simulink model "interpretar_ensaios"  (R2012b)
settings: Solver=ode3  StartTime=0.0  StopTime=4.9999  FixedStep=1e-4  MaxStep=1e-4  RelTol=1e-3
libraries: simulink x3, Encoder x1
settings Model: Creator=h3now  LastModifiedBy=h3now

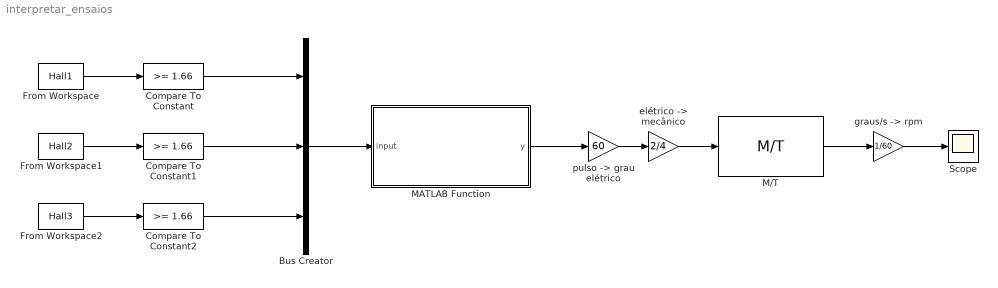
== system interpretar_ensaios ==
  Bus Creator : BusCreator  Inputs=3
  Compare To Constant : simulink/Logic and Bit Operations/Compare To Constant  relop=>=  const=1.66  OutDataTypeStr=uint8
  Compare To Constant1 : simulink/Logic and Bit Operations/Compare To Constant  relop=>=  const=1.66  OutDataTypeStr=uint8
  Compare To Constant2 : simulink/Logic and Bit Operations/Compare To Constant  relop=>=  const=1.66  OutDataTypeStr=uint8
  From Workspace : FromWorkspace  VariableName=Hall1  SampleTime=0  OutputAfterFinalValue=Holding final value
  From Workspace1 : FromWorkspace  VariableName=Hall2  SampleTime=0
  From Workspace2 : FromWorkspace  VariableName=Hall3  SampleTime=0
  M/T : Encoder/M//T  Ts=0.01
  MATLAB Function : MATLAB Function  TreatAsAtomicUnit=on
  Scope : Scope
      settings: SaveName=vel  SampleInput=on
  "elétrico -> mecânico" : Gain  Gain=2/4
  "graus/s -> rpm" : Gain  Gain=1/60
  "pulso -> grau elétrico" : Gain  Gain=60
  wires:
  Bus Creator/1 -> MATLAB Function/1(input)
  From Workspace/1 -> Compare To Constant/1
  From Workspace1/1 -> Compare To Constant1/1
  From Workspace2/1 -> Compare To Constant2/1
  Compare To Constant/1 -> Bus Creator/1
  Compare To Constant1/1 -> Bus Creator/2
  Compare To Constant2/1 -> Bus Creator/3
  MATLAB Function/1(y) -> "pulso -> grau elétrico"/1
  "pulso -> grau elétrico"/1 -> "elétrico -> mecânico"/1
  "elétrico -> mecânico"/1 -> M/T/1
  M/T/1 -> "graus/s -> rpm"/1
  "graus/s -> rpm"/1 -> Scope/1

== matlab function interpretar_ensaios/MATLAB Function ==
  data: y output; input input
function y = state_machine(input)
%#codegen

% Initializing persistent variables.
persistent theta;
persistent state;
if isempty(theta)
    % 'theta' stores the angular position.
    theta = 0; 
    
    % check starting state and store it in 'state'.
    if isequal(input, [0,0,1]')
        state = 0;
    elseif isequal(input, [1,0,1]')
        state = 1;
    elseif isequal(input, [1,0,0]')
        state = 2;
    elseif isequal(input, [1,1,0]')
        state = 3;
    elseif isequal(input, [0,1,0]')
        state = 4;
    elseif isequal(input, [0,1,1]')
        state = 5;
    else
        state = -1;
    end
        
end

% State machine.
switch state
    case 0
        % keep state.
        if isequal(input,[0,0,1]')
        % go to next state.
        elseif isequal(input,[1,0,1]')
            state = 1;
            theta = theta + 1;
        % go to previous state.
        elseif isequal(input,[0,1,1]')
            state = 5;
            theta = theta - 1;
        % go to error state.
        else
            state = -1;
        end
        
    case 1
        % keep state.
        if isequal(input,[1,0,1]')
        % go to next state.
        elseif isequal(input,[1,0,0]')
            state = 2;
            theta = theta + 1;
        % go to previous state.
        elseif isequal(input,[0,0,1]')
            state = 0;
            theta = theta - 1;
        % go to error state.
        else
            state = -1;
        end
        
    case 2
        % keep state.
        if isequal(input,[1,0,0]')
        % go to next state.
        elseif isequal(input,[1,1,0]')
            state = 3;
            theta = theta + 1;
        % go to previous state.
        elseif isequal(input,[1,0,1]')
            state = 1;
            theta = theta - 1;
        % go to error state.
        else
            state = -1;
        end
        
    case 3
        % keep state.
        if isequal(input,[1,1,0]')
        % go to next state.
        elseif isequal(input,[0,1,0]')
            state = 4;
            theta = theta + 1;
        % go to previous state.
        elseif isequal(input,[1,0,0]')
            state = 2;
            theta = theta - 1;
        % go to error state.
        else
            state = -1;
        end
        
    case 4
        % keep state.
        if isequal(input,[0,1,0]')
        % go to next state.
        elseif isequal(input,[0,1,1]')
            state = 5;
            theta = theta + 1;
        % go to previous state.
        elseif isequal(input,[1,1,0]')
            state = 3;
            theta = theta - 1;
        % go to error state.
        else
            state = -1;
        end
        
    case 5
        % keep state.
        if isequal(input,[0,1,1]')
        % go to next state.
        elseif isequal(input,[0,0,1]')
            state = 0;
            theta = theta + 1;
        % go to previous state.
        elseif isequal(input,[0,1,0]')
            state = 4;
            theta = theta - 1;
        % go to error state.
        else
            state = -1;
        end
            
end

% Output
y = theta;
